simulink model "Exp8_ADM"  (R2026a)
settings: Solver=VariableStepAuto  StopTime=1
settings Model: Creator=yatha  LastModifiedBy=yatha

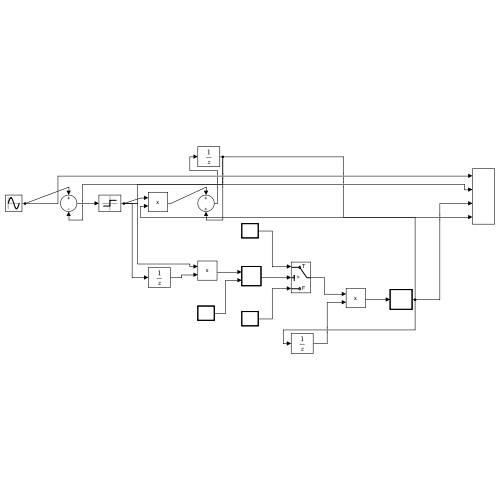
[thumbnail: Simulink's stored preview of the top-level diagram]
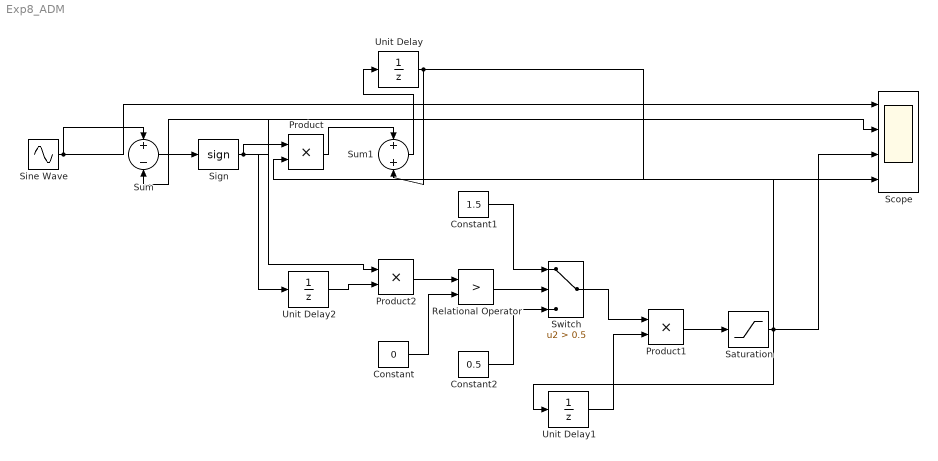
== system Exp8_ADM ==
  Constant : Constant  Value=0
  Constant1 : Constant  Value=1.5
  Constant2 : Constant  Value=0.5
  Product : Product
  Product1 : Product
  Product2 : Product
  Relational Operator : RelationalOperator  Operator=>  OutDataTypeStr=boolean  RndMeth=Simplest  InputSameDT=off
  Saturation : Saturate  UpperLimit=2  LowerLimit=0.1
  Scope : Scope  NumInputPorts=4
  Sign : Signum
  Sine Wave : Sin  Amplitude=5  Frequency=12.5664  SampleTime=0
  Sum : Sum  Inputs=+-
  Sum1 : Sum
  Switch : Switch  Criteria=u2 > Threshold  Threshold=0.5  SaturateOnIntegerOverflow=off  InputSameDT=off
  Unit Delay : UnitDelay  SampleTime=0.05
  Unit Delay1 : UnitDelay  InitialCondition=0.5  SampleTime=0.05
  Unit Delay2 : UnitDelay  SampleTime=0.05
  wires:
  Sine Wave/1 -> Sum/1, Scope/1
  Sum/1 -> Sign/1
  Sign/1 -> Product/1, Unit Delay2/1, Product2/1, Scope/2
  Saturation/1 -> Product/2, Unit Delay1/1, Scope/3
  Product/1 -> Sum1/1
  Sum1/1 -> Unit Delay/1
  Unit Delay/1 -> Sum1/2, Sum/2, Scope/4
  Unit Delay2/1 -> Product2/2
  Product2/1 -> Relational Operator/1
  Constant/1 -> Relational Operator/2
  Constant1/1 -> Switch/1
  Relational Operator/1 -> Switch/2
  Constant2/1 -> Switch/3
  Switch/1 -> Product1/1
  Unit Delay1/1 -> Product1/2
  Product1/1 -> Saturation/1
